simulink model "full_system"  (R2022b)
settings: Solver=VariableStepAuto  StartTime=0.0  StopTime=60  RelTol=1e-3
model workspace (MAT data in the model file):
  J_left = Simulink.Parameter
  J_left.Value = 0.0896732223267
  J_left.Description = 'left wheel inertia'
  J_left.DataType = 'auto'
  J_left.Complexity = 'real'
  J_left.Dimensions = [1 1]
  J_right = Simulink.Parameter
  J_right.Value = 0.0740595319322
  J_right.Description = 'right wheel inertia'
  J_right.DataType = 'auto'
  J_right.Complexity = 'real'
  J_right.Dimensions = [1 1]
  K_L = Simulink.Parameter
  K_L.Value = Simulink.data.Expression
  K_L.Value.ExpressionString = "1.2108*K_R"
  K_L.DataType = 'auto'
  K_L.Complexity = 'real'
  K_L.Dimensions = -1
  K_R = Simulink.Parameter
  K_R.Value = 2.0947
  K_R.DataType = 'auto'
  K_R.Complexity = 'real'
  K_R.Dimensions = [1 1]
  K_w = Simulink.Parameter
  K_w.Value = 4
  K_w.Description = 'heading controller gain'
  K_w.DataType = 'auto'
  K_w.Complexity = 'real'
  K_w.Dimensions = [1 1]
  T_max = Simulink.Parameter
  T_max.Value = 10
  T_max.Description = 'maximum allowable torque command'
  T_max.DataType = 'auto'
  T_max.DocUnits = 'N*m'
  T_max.Complexity = 'real'
  T_max.Dimensions = [1 1]
  bw = Simulink.Parameter
  bw.Value = 0.24
  bw.Description = 'Distance between the two drive wheels'
  bw.DataType = 'auto'
  bw.DocUnits = 'm'
  bw.Complexity = 'real'
  bw.Dimensions = [1 1]
  r_turn = Simulink.Parameter
  r_turn.Value = 0.2
  r_turn.Description = 'Minimum turn radius of the car'
  r_turn.DataType = 'auto'
  r_turn.Min = 0
  r_turn.DocUnits = 'm'
  r_turn.Complexity = 'real'
  r_turn.Dimensions = [1 1]
  r_wheel = Simulink.Parameter
  r_wheel.Value = 0.11
  r_wheel.Description = 'Wheel radius'
  r_wheel.DataType = 'auto'
  r_wheel.DocUnits = 'm'
  r_wheel.Complexity = 'real'
  r_wheel.Dimensions = [1 1]
  v_base = Simulink.Parameter
  v_base.Value = 0.8
  v_base.Description = 'base wheel speed (m/s) used for turns
    | v_base = w_turn_max * bw/2'
  v_base.DataType = 'auto'
  v_base.DocUnits = 'm/s'
  v_base.Complexity = 'real'
  v_base.Dimensions = [1 1]
  v_max = Simulink.Parameter
  v_max.Value = 1
  v_max.Description = 'max car speed in m/s'
  v_max.DataType = 'auto'
  v_max.DocUnits = 'm/s'
  v_max.Complexity = 'real'
  v_max.Dimensions = [1 1]
  w_max = Simulink.Parameter
  w_max.Value = Simulink.data.Expression
  w_max.Value.ExpressionString = "9.0909*v_max"
  w_max.Description = 'max wheel speed in rad/s
    | w_max = v_max/r_wheel'
  w_max.DataType = 'auto'
  w_max.DocUnits = 'rad/s'
  w_max.Complexity = 'real'
  w_max.Dimensions = -1
  w_turn_max = Simulink.Parameter
  w_turn_max.Value = 4
  w_turn_max.Description = 'max turning speed of car in rad/s
    | w_turn_max = w_max * r_wheel/bw'
  w_turn_max.DataType = 'auto'
  w_turn_max.DocUnits = 'rad/s'
  w_turn_max.Complexity = 'real'
  w_turn_max.Dimensions = [1 1]
values from neighbouring files (symbols this model uses):
  J_left = 0.089673222326686    (= 0.0896732223267)    [calc_torque_gains.m]
  J_right = 0.074059531932167    (= 0.0740595319322)    [calc_torque_gains.m]
undefined symbols (not defined in the file or in its folder): duration, effort, index, joint_name, K_l, K_r, left_wheel_hinge, model_name, pioneer2dx, right_wheel_hinge
libraries: robotgazebolib x46, simulink x4, robotcorelib x2, SignalEditorBlockLib x1
settings Model: Creator=22546723@sun.ac.za  LastModifiedBy=22546723@sun.ac.za

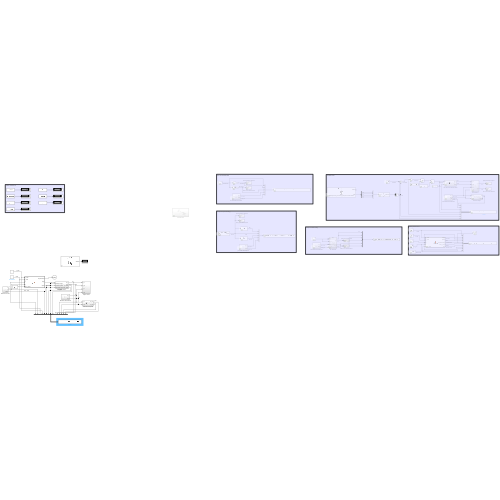
[thumbnail: Simulink's stored preview of the top-level diagram]
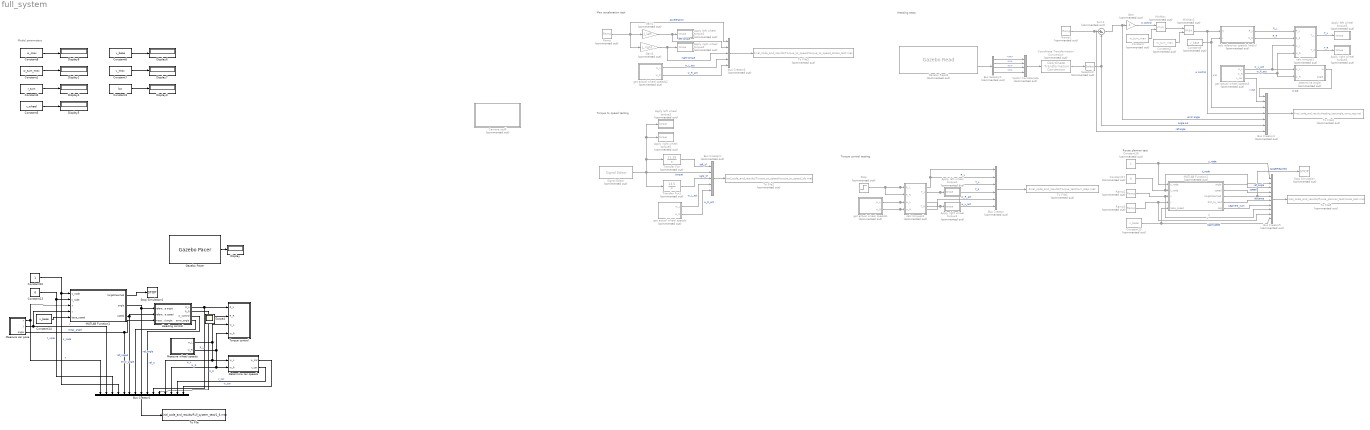
== system full_system ==
  note: Route planner test
  note: Heading tests
  note: Torque control testing
  note: Max acceleration test
  note: Torque to speed testing
  note: Model parameters
  Apply left wheel torque1 : Subsystem  Commented=on
  Apply left wheel torque2 : Subsystem  Commented=on
  Apply left wheel torque3 : Subsystem  Commented=on
  Apply left wheel torque5 : Subsystem  Commented=on
  Apply right wheel torque1 : Subsystem  Commented=on
  Apply right wheel torque2 : Subsystem  Commented=on
  Apply right wheel torque3 : Subsystem  Commented=on
  Apply right wheel torque5 : Subsystem  Commented=on
  Bus Creator : BusCreator  Commented=on  Inputs=6
  Bus Creator1 : BusCreator  Inputs=15
  Bus Creator2 : BusCreator  Commented=on  Inputs=5
  Bus Creator3 : BusCreator  Commented=on  Inputs=5
  Bus Creator4 : BusCreator  Commented=on  Inputs=7
  Bus Creator5 : BusCreator  Commented=on  Inputs=10
  Bus Selector1 : BusSelector  Commented=on  OutputSignals=orientation.w,orientation.x,orientation.y,orientation.z
  Camera stuff : Subsystem  Commented=on
  Constant : Constant  Commented=on  Value=w_turn_max
  Constant1 : Constant  Value=w_turn_max
  Constant10 : Constant
  Constant13 : Constant  Value=6
  Constant14 : Constant  Value=v_base
  Constant15 : Constant  Commented=on  Value=v_base
  Constant16 : Constant  Commented=on
  Constant17 : Constant  Commented=on  Value=8
  Constant2 : Constant  Commented=on  Value=-w_turn_max
  Constant3 : Constant  Value=bw
  Constant4 : Constant  Value=r_turn
  Constant5 : Constant  Value=r_wheel
  Constant6 : Constant  Value=v_base
  Constant7 : Constant  Value=v_max
  Constant8 : Constant  Value=w_max
  Constant9 : Constant  Commented=on  Value=v_base
  Coordinate Transformation Conversion : robotcorelib/Coordinate Transformation Conversion  Commented=on  InputRepresentation=Quaternion  InputEulerSequence=ZYX  ShowTrVecInputPort=on  OutputRepresentation=Euler Angles  OutputEulerSequence=ZYX  ShowTrVecOutputPort=on  SimulateUsing=Interpreted execution
  Determine car speeds : Subsystem
  Display{,2..8} (8 alike) : Display
  Gain : Gain  Commented=on  Gain=4
  Gain2 : Gain  Commented=on  Gain=J_left
  Gain3 : Gain  Commented=on  Gain=J_right
  Gazebo Pacer : robotgazebolib/Gazebo Pacer  ResetBehavior=Reset Gazebo simulation time  SampleTime=0.001
  Gazebo Read4 : robotgazebolib/Gazebo Read  Commented=on  topicSource=From Gazebo  topic=/gazebo/ground_truth/world_pose/pioneer2dx/chassis  messageType=gazebo_msgs/Pose  sampleTime=0.001  fixedAxisBusStatus=off  jointAxisCount=2
  Heading control : Subsystem
  MATLAB Function1 : MATLAB Function  TreatAsAtomicUnit=on
  MATLAB Function2 : MATLAB Function  Commented=on  TreatAsAtomicUnit=on
  Measure car pose : Subsystem
  Measure wheel speeds : Subsystem
  MinMax : MinMax  Commented=on  Inputs=2
  MinMax1 : MinMax  Commented=on  Function=max  Inputs=2
  Ramp : simulink/Sources/Ramp  Commented=on  slope=1  start=0  InitialOutput=0
  Ramp1 : simulink/Sources/Ramp  Commented=on  slope=-1  start=0  InitialOutput=0
  Ramp2 : simulink/Sources/Ramp  Commented=on  slope=8/16.7  start=0  InitialOutput=0
  Ramp3 : simulink/Sources/Ramp  Commented=on  slope=1/16.7  start=0  InitialOutput=0
  Selector2 : Selector  Commented=on  InputPortWidth=3  IndexOptions=Index vector (dialog)  Indices=1  OutputSizes=1
  Signal Editor : SignalEditorBlockLib/Signal Editor  Commented=on  FileName=test_signals.mat  ActiveScenario=torque_to_speed  ActiveSignal=torque  IsBus=off  OutputBusObjectStr=Bus: BusObject  SampleTime=0  Interpolate=off  ZeroCross=off  OutputAfterFinalValue=Setting to zero  Unit=inherit  PreserveSignalName=on
  Step : Step  Commented=on  Time=0  After=4  SampleTime=0
  Stop Simulation : Stop  Commented=on
  Stop Simulation1 : Stop
  Sum1 : Sum  Commented=on  Inputs=|+-
  To File : ToFile  Filename=Final_code_and_results/Full_system_test/1_6.mat  MatrixName=data  SaveFormat=Timeseries
  To File1 : ToFile  Commented=on  Filename=Final_code_and_results/Torque_test/turn_step.mat  MatrixName=data  SaveFormat=Timeseries
  To File2 : ToFile  Commented=on  Filename=Final_code_and_results/Torque_to_speed/torque_to_speed_tfs.mat  MatrixName=data  SaveFormat=Timeseries
  To File3 : ToFile  Commented=on  Filename=Final_code_and_results/Torque_to_speed/torque_to_speed_stress_test.mat  MatrixName=data  SaveFormat=Timeseries
  To File4 : ToFile  Commented=on  Filename=Final_code_and_results/Heading_test/angle_ramp_neg.mat  MatrixName=data  SaveFormat=Timeseries
  To File5 : ToFile  Commented=on  Filename=Final_code_and_results/Route_planner_test/route_test.mat  MatrixName=data  SaveFormat=Timeseries
  Torque control : Subsystem
  Transfer Fcn : TransferFcn  Commented=on  Numerator=11.15  Denominator=[1 0]
  Transfer Fcn1 : TransferFcn  Commented=on  Numerator=13.5  Denominator=[1 0]
  Vector Concatenate : Concatenate  Commented=on  NumInputs=4
  calc reference speeds (rad/s) : Subsystem  Commented=on
  calc torques1 : Subsystem  Commented=on
  calc torques3 : Subsystem  Commented=on
  determine angle : Subsystem  Commented=on
  get actual wheel speeds : Subsystem  Commented=on
  get actual wheel speeds1 : Subsystem  Commented=on
  get actual wheel speeds2 : Subsystem  Commented=on
  get actual wheel speeds3 : Subsystem  Commented=on
  Scope4 : Scope
  wires:
  Gazebo Pacer/1 -> Display/1
  Constant1/1 -> Display2/1
  Constant3/1 -> Display3/1
  Constant4/1 -> Display4/1
  Constant5/1 -> Display5/1
  Constant6/1 -> Display6/1
  Constant7/1 -> Display7/1
  Constant8/1 -> Display8/1
  Constant10/1 -> MATLAB Function1/1(s_node), Bus Creator1/4  "s_node"
  Constant13/1 -> MATLAB Function1/2(t_node), Bus Creator1/3  "t_node"
  Constant14/1 -> MATLAB Function1/5(base_speed)
  Signal Editor/1 -> Apply left wheel torque5/1(torque), Apply right wheel torque5/1(torque), Transfer Fcn/1, Bus Creator2/2, Transfer Fcn1/1  "torque"
  Bus Creator2/1 -> To File2/1
  Transfer Fcn/1 -> Bus Creator2/1  "left_tf"
  Transfer Fcn1/1 -> Bus Creator2/3  "right_tf"
  get actual wheel speeds/1(w_L) -> Bus Creator2/4  "w_L_act"
  get actual wheel speeds/2(w_R) -> Bus Creator2/5  "w_R_act"
  get actual wheel speeds1/1(w_L) -> Bus Creator/6, calc torques3/3(w_L)  "w_L_act"
  get actual wheel speeds1/2(w_R) -> Bus Creator/5, calc torques3/4(w_R)  "w_R_act"
  calc torques3/2(T_R) -> Bus Creator/4, Apply right wheel torque1/1(torque)  "T_R"
  calc torques3/1(T_L) -> Bus Creator/3, Apply left wheel torque1/1(torque)  "T_L"
  Step/1 -> Bus Creator/1, Bus Creator/2, calc torques3/1(R_L), calc torques3/2(R_R)  "R_L"
  Bus Creator/1 -> To File1/1
  Gain3/1 -> Apply right wheel torque2/1(torque), Bus Creator3/3  "right torque"
  Gain2/1 -> Apply left wheel torque2/1(torque), Bus Creator3/2  "left torque"
  Ramp/1 -> Gain3/1, Gain2/1, Bus Creator3/1  "acceleration"
  get actual wheel speeds2/2(w_R) -> Bus Creator3/5  "w_R_act"
  get actual wheel speeds2/1(w_L) -> Bus Creator3/4  "w_L_act"
  Bus Creator3/1 -> To File3/1
  Gain/1 -> MinMax/1  "w control"
  Constant2/1 -> MinMax1/2
  MinMax/1 -> MinMax1/1
  Constant/1 -> MinMax/2
  Sum1/1 -> Bus Creator4/5, Gain/1  "error angle"
  Selector2/1 -> Bus Creator4/6, Sum1/2  "angle out"
  Gazebo Read4/2 -> Bus Selector1/1
  Coordinate Transformation Conversion/1 -> Selector2/1
  Bus Selector1/4 -> Vector Concatenate/4  "<z>"
  Bus Selector1/3 -> Vector Concatenate/3  "<y>"
  Bus Selector1/1 -> Vector Concatenate/1  "<w>"
  Bus Selector1/2 -> Vector Concatenate/2  "<x>"
  Vector Concatenate/1 -> Coordinate Transformation Conversion/1
  get actual wheel speeds3/1(w_L) -> determine angle/1(w_L), calc torques1/3(w_L)  "w_L_act"
  calc reference speeds (rad/s)/1(R_L) -> calc torques1/1(R_L)  "R_L"
  calc reference speeds (rad/s)/2(R_R) -> calc torques1/2(R_R)  "R_R"
  Ramp1/1 -> Bus Creator4/7, Sum1/1  "ref angle"
  calc torques1/2(T_R) -> Apply right wheel torque3/1(torque)  "T_R"
  MinMax1/1 -> calc reference speeds (rad/s)/1(w), Bus Creator4/4  "w control"
  get actual wheel speeds3/2(w_R) -> determine angle/2(w_R), calc torques1/4(w_R)  "w_R_act"
  calc torques1/1(T_L) -> Apply left wheel torque3/1(torque)  "T_L"
  Constant9/1 -> Bus Creator4/3, calc reference speeds (rad/s)/2(v)  "v in"
  Bus Creator4/1 -> To File4/1
  determine angle/1(w) -> Bus Creator4/1  "w out"
  get actual wheel speeds3/3(v_car) -> Bus Creator4/2  "v out"
  Constant15/1 -> MATLAB Function2/5(base_speed), Bus Creator5/10  "base speed"
  Ramp3/1 -> MATLAB Function2/4(y), Bus Creator5/9  "y"
  Ramp2/1 -> Bus Creator5/8, MATLAB Function2/3(x)  "x"
  Constant17/1 -> Bus Creator5/2, MATLAB Function2/2(t_node)  "t_node"
  Constant16/1 -> MATLAB Function2/1(s_node), Bus Creator5/1  "s_node"
  MATLAB Function2/1(angle) -> Bus Creator5/3  "ref_angle"
  MATLAB Function2/2(speed) -> Bus Creator5/4  "speed"
  MATLAB Function2/3(targetReached) -> Bus Creator5/5, Stop Simulation/1  "targetReached"
  MATLAB Function2/4(dist_to_next) -> Bus Creator5/6  "distance"
  MATLAB Function2/5(seg) -> Bus Creator5/7  "segment_num"
  Bus Creator5/1 -> To File5/1
  MATLAB Function1/1(targetReached) -> Stop Simulation1/1
  Measure wheel speeds/1(w_L) -> Bus Creator1/12, Determine car speeds/1(w_L), Torque control/3(w_L)  "w_L"
  Measure wheel speeds/2(w_R) -> Bus Creator1/13, Determine car speeds/2(w_R), Torque control/4(w_R)  "w_R"
  MATLAB Function1/2(angle) -> Heading control/1(reference angle), Bus Creator1/8  "ref_angle"
  MATLAB Function1/3(speed) -> Heading control/2(reference speed), Bus Creator1/6  "ref_speed"
  Heading control/1(R_L) -> Bus Creator1/10, Torque control/1(R_L)  "R_L"
  Heading control/2(R_R) -> Bus Creator1/11, Torque control/2(R_R)  "R_R"
  Measure car pose/3(angle) -> Heading control/3(measured angle), Bus Creator1/5  "meas_angle"
  Measure car pose/1(x) -> MATLAB Function1/3(x), Bus Creator1/1  "x"
  Measure car pose/2(y) -> MATLAB Function1/4(y), Bus Creator1/2  "y"
  Determine car speeds/1(w_car) -> Bus Creator1/15  "w_car"
  Determine car speeds/2(v_car) -> Bus Creator1/14  "v_car"
  Bus Creator1/1 -> To File/1
  Heading control/3(w_control) -> Bus Creator1/9  "ref_w"
  Heading control/4(error_angle) -> Bus Creator1/7  "error_angle"

== system full_system/Apply left wheel torque1 ==
  torque : Inport  SampleTime=0.001
  Bus Assignment : BusAssignment  AssignedSignals=model_name,joint_name,index,effort,duration.nano_seconds
  Constant : Constant  Value=0  OutDataTypeStr=uint32  SampleTime=0.001
  Constant1 : Constant  Value=1e7  SampleTime=0.001
  Gazebo Apply Command : robotgazebolib/Gazebo Apply Command  cmdType=ApplyJointTorque  sampleTime=0.001
  Gazebo Blank Message : robotgazebolib/Gazebo Blank Message  msgType=ApplyJointTorque  sampleTime=0.001  busName='Gazebo_SL_Bus_gazebo_msgs_ApplyJointTorque'
  Gazebo Select Entity : robotgazebolib/Gazebo Select Entity  modelElemName=pioneer2dx/left_wheel_hinge  outputArraySize=128  OutputLabel=Joint  SelectType=Joint
  wires:
  Gazebo Select Entity/1 -> Bus Assignment/2
  Bus Assignment/1 -> Gazebo Apply Command/1
  Gazebo Blank Message/1 -> Bus Assignment/1
  Constant/1 -> Bus Assignment/4
  Gazebo Select Entity/2 -> Bus Assignment/3
  Constant1/1 -> Bus Assignment/6
  torque/1 -> Bus Assignment/5

== system full_system/Apply left wheel torque2 ==
  torque : Inport  SampleTime=0.001
  Bus Assignment : BusAssignment  AssignedSignals=model_name,joint_name,index,effort,duration.nano_seconds
  Constant : Constant  Value=0  OutDataTypeStr=uint32  SampleTime=0.001
  Constant1 : Constant  Value=1e7  SampleTime=0.001
  Gazebo Apply Command : robotgazebolib/Gazebo Apply Command  cmdType=ApplyJointTorque  sampleTime=0.001
  Gazebo Blank Message : robotgazebolib/Gazebo Blank Message  msgType=ApplyJointTorque  sampleTime=0.001  busName='Gazebo_SL_Bus_gazebo_msgs_ApplyJointTorque'
  Gazebo Select Entity : robotgazebolib/Gazebo Select Entity  modelElemName=pioneer2dx/left_wheel_hinge  outputArraySize=128  OutputLabel=Joint  SelectType=Joint
  wires:
  Gazebo Select Entity/1 -> Bus Assignment/2
  Bus Assignment/1 -> Gazebo Apply Command/1
  Gazebo Blank Message/1 -> Bus Assignment/1
  Constant/1 -> Bus Assignment/4
  Gazebo Select Entity/2 -> Bus Assignment/3
  Constant1/1 -> Bus Assignment/6
  torque/1 -> Bus Assignment/5

== system full_system/Apply left wheel torque3 ==
  torque : Inport  SampleTime=0.001
  Bus Assignment : BusAssignment  AssignedSignals=model_name,joint_name,index,effort,duration.nano_seconds
  Constant : Constant  Value=0  OutDataTypeStr=uint32  SampleTime=0.001
  Constant1 : Constant  Value=1e7  SampleTime=0.001
  Gazebo Apply Command : robotgazebolib/Gazebo Apply Command  cmdType=ApplyJointTorque  sampleTime=0.001
  Gazebo Blank Message : robotgazebolib/Gazebo Blank Message  msgType=ApplyJointTorque  sampleTime=0.001  busName='Gazebo_SL_Bus_gazebo_msgs_ApplyJointTorque'
  Gazebo Select Entity : robotgazebolib/Gazebo Select Entity  modelElemName=pioneer2dx/left_wheel_hinge  outputArraySize=128  OutputLabel=Joint  SelectType=Joint
  wires:
  Gazebo Select Entity/1 -> Bus Assignment/2
  Bus Assignment/1 -> Gazebo Apply Command/1
  Gazebo Blank Message/1 -> Bus Assignment/1
  Constant/1 -> Bus Assignment/4
  Gazebo Select Entity/2 -> Bus Assignment/3
  Constant1/1 -> Bus Assignment/6
  torque/1 -> Bus Assignment/5

== system full_system/Apply left wheel torque5 ==
  torque : Inport  SampleTime=0.001
  Bus Assignment : BusAssignment  AssignedSignals=model_name,joint_name,index,effort,duration.nano_seconds
  Constant : Constant  Value=0  OutDataTypeStr=uint32  SampleTime=0.001
  Constant1 : Constant  Value=1e7  SampleTime=0.001
  Gazebo Apply Command : robotgazebolib/Gazebo Apply Command  cmdType=ApplyJointTorque  sampleTime=0.001
  Gazebo Blank Message : robotgazebolib/Gazebo Blank Message  msgType=ApplyJointTorque  sampleTime=0.001  busName='Gazebo_SL_Bus_gazebo_msgs_ApplyJointTorque'
  Gazebo Select Entity : robotgazebolib/Gazebo Select Entity  modelElemName=pioneer2dx/left_wheel_hinge  outputArraySize=128  OutputLabel=Joint  SelectType=Joint
  wires:
  Gazebo Select Entity/1 -> Bus Assignment/2
  Bus Assignment/1 -> Gazebo Apply Command/1
  Gazebo Blank Message/1 -> Bus Assignment/1
  Constant/1 -> Bus Assignment/4
  Gazebo Select Entity/2 -> Bus Assignment/3
  Constant1/1 -> Bus Assignment/6
  torque/1 -> Bus Assignment/5

== system full_system/Apply right wheel torque1 ==
  torque : Inport  SampleTime=0.001
  Bus Assignment : BusAssignment  AssignedSignals=model_name,joint_name,index,effort,duration.nano_seconds
  Constant : Constant  Value=0  OutDataTypeStr=uint32  SampleTime=0.001
  Constant1 : Constant  Value=1e7  SampleTime=0.001
  Gazebo Apply Command : robotgazebolib/Gazebo Apply Command  cmdType=ApplyJointTorque  sampleTime=0.001
  Gazebo Blank Message : robotgazebolib/Gazebo Blank Message  msgType=ApplyJointTorque  sampleTime=0.001  busName='Gazebo_SL_Bus_gazebo_msgs_ApplyJointTorque'
  Gazebo Select Entity : robotgazebolib/Gazebo Select Entity  modelElemName=pioneer2dx/right_wheel_hinge  outputArraySize=128  OutputLabel=Joint  SelectType=Joint
  wires:
  Gazebo Select Entity/1 -> Bus Assignment/2
  Bus Assignment/1 -> Gazebo Apply Command/1
  Gazebo Blank Message/1 -> Bus Assignment/1
  Constant/1 -> Bus Assignment/4
  Gazebo Select Entity/2 -> Bus Assignment/3
  Constant1/1 -> Bus Assignment/6
  torque/1 -> Bus Assignment/5

== system full_system/Apply right wheel torque2 ==
  torque : Inport  SampleTime=0.001
  Bus Assignment : BusAssignment  AssignedSignals=model_name,joint_name,index,effort,duration.nano_seconds
  Constant : Constant  Value=0  OutDataTypeStr=uint32  SampleTime=0.001
  Constant1 : Constant  Value=1e7  SampleTime=0.001
  Gazebo Apply Command : robotgazebolib/Gazebo Apply Command  cmdType=ApplyJointTorque  sampleTime=0.001
  Gazebo Blank Message : robotgazebolib/Gazebo Blank Message  msgType=ApplyJointTorque  sampleTime=0.001  busName='Gazebo_SL_Bus_gazebo_msgs_ApplyJointTorque'
  Gazebo Select Entity : robotgazebolib/Gazebo Select Entity  modelElemName=pioneer2dx/right_wheel_hinge  outputArraySize=128  OutputLabel=Joint  SelectType=Joint
  wires:
  Gazebo Select Entity/1 -> Bus Assignment/2
  Bus Assignment/1 -> Gazebo Apply Command/1
  Gazebo Blank Message/1 -> Bus Assignment/1
  Constant/1 -> Bus Assignment/4
  Gazebo Select Entity/2 -> Bus Assignment/3
  Constant1/1 -> Bus Assignment/6
  torque/1 -> Bus Assignment/5

== system full_system/Apply right wheel torque3 ==
  torque : Inport  SampleTime=0.001
  Bus Assignment : BusAssignment  AssignedSignals=model_name,joint_name,index,effort,duration.nano_seconds
  Constant : Constant  Value=0  OutDataTypeStr=uint32  SampleTime=0.001
  Constant1 : Constant  Value=1e7  SampleTime=0.001
  Gazebo Apply Command : robotgazebolib/Gazebo Apply Command  cmdType=ApplyJointTorque  sampleTime=0.001
  Gazebo Blank Message : robotgazebolib/Gazebo Blank Message  msgType=ApplyJointTorque  sampleTime=0.001  busName='Gazebo_SL_Bus_gazebo_msgs_ApplyJointTorque'
  Gazebo Select Entity : robotgazebolib/Gazebo Select Entity  modelElemName=pioneer2dx/right_wheel_hinge  outputArraySize=128  OutputLabel=Joint  SelectType=Joint
  wires:
  Gazebo Select Entity/1 -> Bus Assignment/2
  Bus Assignment/1 -> Gazebo Apply Command/1
  Gazebo Blank Message/1 -> Bus Assignment/1
  Constant/1 -> Bus Assignment/4
  Gazebo Select Entity/2 -> Bus Assignment/3
  Constant1/1 -> Bus Assignment/6
  torque/1 -> Bus Assignment/5

== system full_system/Apply right wheel torque5 ==
  torque : Inport  SampleTime=0.001
  Bus Assignment : BusAssignment  AssignedSignals=model_name,joint_name,index,effort,duration.nano_seconds
  Constant : Constant  Value=0  OutDataTypeStr=uint32  SampleTime=0.001
  Constant1 : Constant  Value=1e7  SampleTime=0.001
  Gazebo Apply Command : robotgazebolib/Gazebo Apply Command  cmdType=ApplyJointTorque  sampleTime=0.001
  Gazebo Blank Message : robotgazebolib/Gazebo Blank Message  msgType=ApplyJointTorque  sampleTime=0.001  busName='Gazebo_SL_Bus_gazebo_msgs_ApplyJointTorque'
  Gazebo Select Entity : robotgazebolib/Gazebo Select Entity  modelElemName=pioneer2dx/right_wheel_hinge  outputArraySize=128  OutputLabel=Joint  SelectType=Joint
  wires:
  Gazebo Select Entity/1 -> Bus Assignment/2
  Bus Assignment/1 -> Gazebo Apply Command/1
  Gazebo Blank Message/1 -> Bus Assignment/1
  Constant/1 -> Bus Assignment/4
  Gazebo Select Entity/2 -> Bus Assignment/3
  Constant1/1 -> Bus Assignment/6
  torque/1 -> Bus Assignment/5

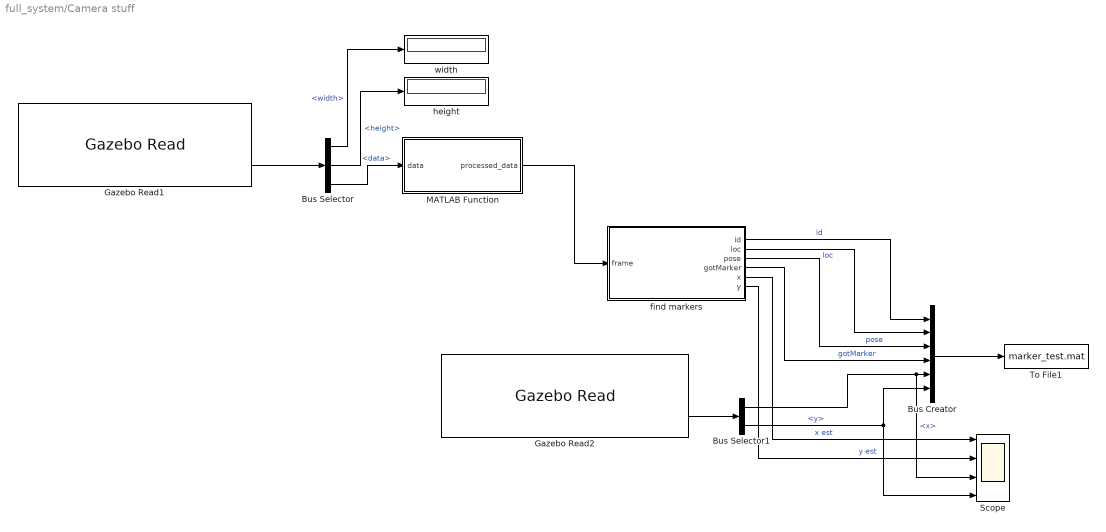
== system full_system/Camera stuff ==
  Bus Creator : BusCreator  Inputs=6
  Bus Selector : BusSelector  OutputSignals=width,height,data
  Bus Selector1 : BusSelector  OutputSignals=position.x,position.y
  Gazebo Read1 : robotgazebolib/Gazebo Read  topicSource=From Gazebo  topic=/gazebo/default/pioneer2dx/camera/camera/image  messageType=gazebo_msgs/Image  sampleTime=0.001  fixedAxisBusStatus=off  jointAxisCount=2
  Gazebo Read2 : robotgazebolib/Gazebo Read  topicSource=From Gazebo  topic=/gazebo/ground_truth/world_pose/pioneer2dx/camera  messageType=gazebo_msgs/Pose  sampleTime=0.001  fixedAxisBusStatus=off  jointAxisCount=2
  MATLAB Function : MATLAB Function  TreatAsAtomicUnit=on
  Scope : Scope  NumInputPorts=4
  To File1 : ToFile  Filename=marker_test.mat  MatrixName=data  SaveFormat=Timeseries
  find markers : MATLAB Function  TreatAsAtomicUnit=on
  height : Display
  width : Display
  wires:
  Bus Creator/1 -> To File1/1
  find markers/3(pose) -> Bus Creator/3  "pose"
  find markers/1(id) -> Bus Creator/1  "id"
  Gazebo Read2/2 -> Bus Selector1/1
  Bus Selector/1 -> width/1  "<width>"
  find markers/6(y) -> Scope/2  "y est"
  find markers/5(x) -> Scope/1  "x est"
  Bus Selector/3 -> MATLAB Function/1(data)  "<data>"
  Bus Selector1/2 -> Scope/4, Bus Creator/6  "<y>"
  find markers/2(loc) -> Bus Creator/2  "loc"
  find markers/4(gotMarker) -> Bus Creator/4  "gotMarker"
  Gazebo Read1/2 -> Bus Selector/1
  Bus Selector/2 -> height/1  "<height>"
  Bus Selector1/1 -> Scope/3, Bus Creator/5  "<x>"
  MATLAB Function/1(processed_data) -> find markers/1(frame)

== system full_system/Determine car speeds ==
  w_L : Inport
  w_R : Inport  Port=2
  Gain2 : Gain  Gain=0.5*r_wheel
  Gain3 : Gain  Gain=r_wheel/bw
  Sum : Sum  Inputs=++|
  Sum4 : Sum  Inputs=|-+
  w_car : Outport
  v_car : Outport  Port=2
  wires:
  Gain3/1 -> w_car/1  "w_turn"
  Sum4/1 -> Gain3/1
  w_R/1 -> Sum4/2, Sum/1
  w_L/1 -> Sum4/1, Sum/2
  Gain2/1 -> v_car/1
  Sum/1 -> Gain2/1

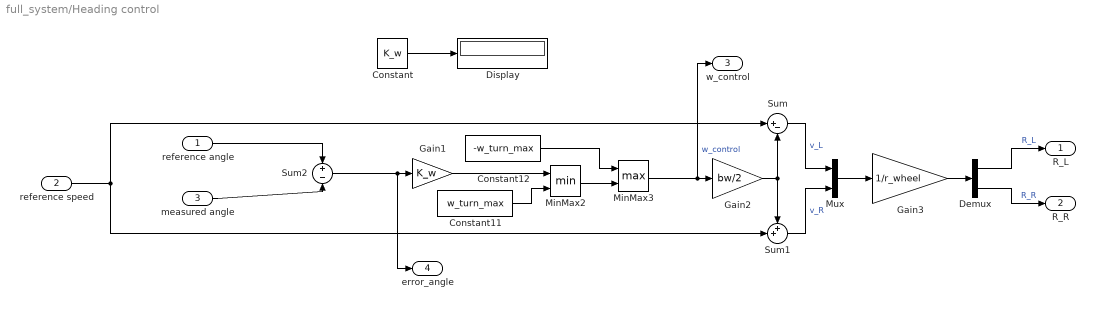
== system full_system/Heading control ==
  reference angle : Inport
  reference speed : Inport  Port=2
  measured angle : Inport  Port=3
  Constant : Constant  Value=K_w
  Constant11 : Constant  Value=w_turn_max
  Constant12 : Constant  Value=-w_turn_max
  Demux : Demux  Outputs=2
  Display : Display
  Gain1 : Gain  Gain=K_w
  Gain2 : Gain  Gain=bw/2
  Gain3 : Gain  Gain=1/r_wheel
  MinMax2 : MinMax  Inputs=2
  MinMax3 : MinMax  Function=max  Inputs=2
  Mux : Mux  Inputs=2
  Sum : Sum  Inputs=|+-
  Sum1 : Sum  Inputs=++|
  Sum2 : Sum  Inputs=+|-
  R_L : Outport
  R_R : Outport  Port=2
  w_control : Outport  Port=3
  error_angle : Outport  Port=4
  wires:
  Constant11/1 -> MinMax2/2
  Demux/2 -> R_R/1  "R_R"
  Constant12/1 -> MinMax3/1
  Gain1/1 -> MinMax2/1
  Demux/1 -> R_L/1  "R_L"
  MinMax2/1 -> MinMax3/2
  MinMax3/1 -> w_control/1, Gain2/1  "w_control"
  Mux/1 -> Gain3/1
  Gain3/1 -> Demux/1
  Sum1/1 -> Mux/2  "v_R"
  Gain2/1 -> Sum1/1, Sum/2
  Sum/1 -> Mux/1  "v_L"
  reference speed/1 -> Sum/1, Sum1/2
  Constant/1 -> Display/1
  Sum2/1 -> error_angle/1, Gain1/1
  reference angle/1 -> Sum2/1
  measured angle/1 -> Sum2/2

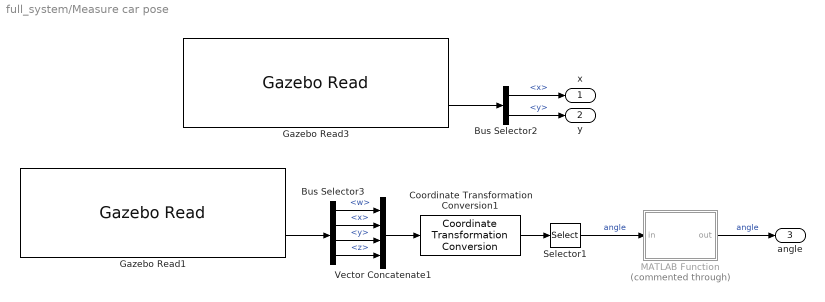
== system full_system/Measure car pose ==
  Bus Selector2 : BusSelector  OutputSignals=position.x,position.y
  Bus Selector3 : BusSelector  OutputSignals=orientation.w,orientation.x,orientation.y,orientation.z
  Coordinate Transformation Conversion1 : robotcorelib/Coordinate Transformation Conversion  InputRepresentation=Quaternion  InputEulerSequence=ZYX  ShowTrVecInputPort=on  OutputRepresentation=Euler Angles  OutputEulerSequence=ZYX  ShowTrVecOutputPort=on  SimulateUsing=Interpreted execution
  Gazebo Read1 : robotgazebolib/Gazebo Read  topicSource=From Gazebo  topic=/gazebo/ground_truth/world_pose/pioneer2dx/chassis  messageType=gazebo_msgs/Pose  sampleTime=0.001  fixedAxisBusStatus=off  jointAxisCount=2
  Gazebo Read3 : robotgazebolib/Gazebo Read  topicSource=From Gazebo  topic=/gazebo/ground_truth/world_pose/pioneer2dx/chassis  messageType=gazebo_msgs/Pose  sampleTime=0.001  fixedAxisBusStatus=off  jointAxisCount=2
  MATLAB Function : MATLAB Function  Commented=through  TreatAsAtomicUnit=on
  Selector1 : Selector  InputPortWidth=3  IndexOptions=Index vector (dialog)  Indices=1  OutputSizes=1
  Vector Concatenate1 : Concatenate  NumInputs=4
  x : Outport
  y : Outport  Port=2
  angle : Outport  Port=3
  wires:
  Coordinate Transformation Conversion1/1 -> Selector1/1
  Vector Concatenate1/1 -> Coordinate Transformation Conversion1/1
  MATLAB Function/1(out) -> angle/1  "angle"
  Bus Selector3/2 -> Vector Concatenate1/2  "<x>"
  Bus Selector2/2 -> y/1  "<y>"
  Bus Selector3/4 -> Vector Concatenate1/4  "<z>"
  Gazebo Read1/2 -> Bus Selector3/1
  Bus Selector3/1 -> Vector Concatenate1/1  "<w>"
  Gazebo Read3/2 -> Bus Selector2/1
  Bus Selector3/3 -> Vector Concatenate1/3  "<y>"
  Bus Selector2/1 -> x/1  "<x>"
  Selector1/1 -> MATLAB Function/1(in)  "angle"

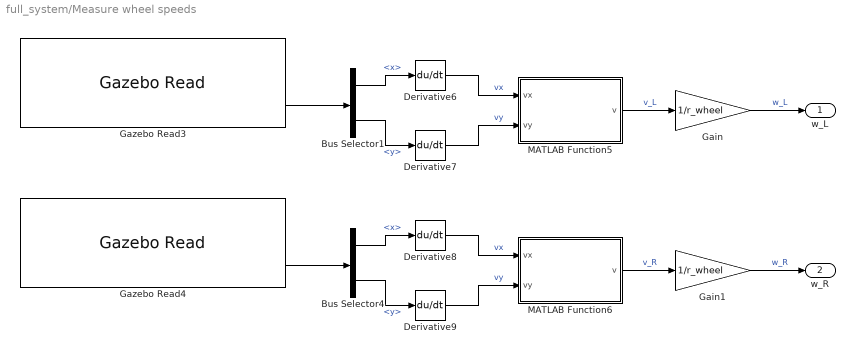
== system full_system/Measure wheel speeds ==
  Bus Selector1 : BusSelector  OutputSignals=position.x,position.y
  Bus Selector4 : BusSelector  OutputSignals=position.x,position.y
  Derivative{6..9} (4 alike) : Derivative
  Gain : Gain  Gain=1/r_wheel
  Gain1 : Gain  Gain=1/r_wheel
  Gazebo Read3 : robotgazebolib/Gazebo Read  topicSource=From Gazebo  topic=/gazebo/ground_truth/world_pose/pioneer2dx/left_wheel  messageType=gazebo_msgs/Pose  sampleTime=0.001  fixedAxisBusStatus=off  jointAxisCount=2
  Gazebo Read4 : robotgazebolib/Gazebo Read  topicSource=From Gazebo  topic=/gazebo/ground_truth/world_pose/pioneer2dx/right_wheel  messageType=gazebo_msgs/Pose  sampleTime=0.001  fixedAxisBusStatus=off  jointAxisCount=2
  MATLAB Function5 : MATLAB Function  TreatAsAtomicUnit=on
  MATLAB Function6 : MATLAB Function  TreatAsAtomicUnit=on
  w_L : Outport
  w_R : Outport  Port=2
  wires:
  Bus Selector4/1 -> Derivative8/1  "<x>"
  Bus Selector4/2 -> Derivative9/1  "<y>"
  Derivative8/1 -> MATLAB Function6/1(vx)  "vx"
  Derivative9/1 -> MATLAB Function6/2(vy)  "vy"
  Derivative6/1 -> MATLAB Function5/1(vx)  "vx"
  Gazebo Read3/2 -> Bus Selector1/1
  Bus Selector1/1 -> Derivative6/1  "<x>"
  Bus Selector1/2 -> Derivative7/1  "<y>"
  Gazebo Read4/2 -> Bus Selector4/1
  Derivative7/1 -> MATLAB Function5/2(vy)  "vy"
  MATLAB Function5/1(v) -> Gain/1  "v_L"
  Gain/1 -> w_L/1  "w_L"
  MATLAB Function6/1(v) -> Gain1/1  "v_R"
  Gain1/1 -> w_R/1  "w_R"

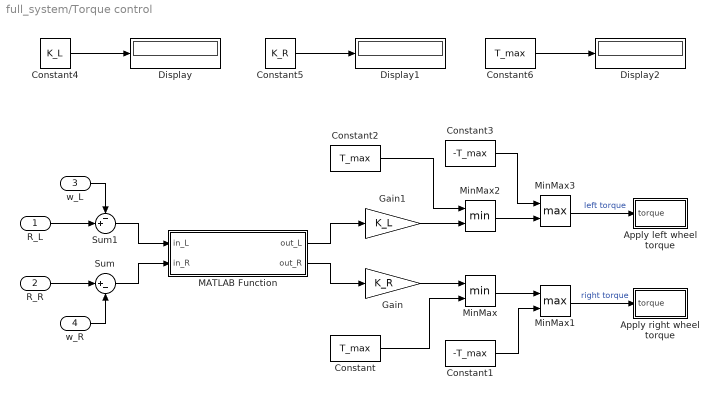
== system full_system/Torque control ==
  R_L : Inport
  R_R : Inport  Port=2
  w_L : Inport  Port=3
  w_R : Inport  Port=4
  Apply left wheel torque : Subsystem
  Apply right wheel torque : Subsystem
  Constant : Constant  Value=T_max
  Constant1 : Constant  Value=-T_max
  Constant2 : Constant  Value=T_max
  Constant3 : Constant  Value=-T_max
  Constant4 : Constant  Value=K_L
  Constant5 : Constant  Value=K_R
  Constant6 : Constant  Value=T_max
  Display : Display
  Display1 : Display
  Display2 : Display
  Gain : Gain  Gain=K_R
  Gain1 : Gain  Gain=K_L
  MATLAB Function : MATLAB Function  TreatAsAtomicUnit=on
  MinMax : MinMax  Inputs=2
  MinMax1 : MinMax  Function=max  Inputs=2
  MinMax2 : MinMax  Inputs=2
  MinMax3 : MinMax  Function=max  Inputs=2
  Sum : Sum  Inputs=|+-
  Sum1 : Sum  Inputs=-+|
  wires:
  Gain/1 -> MinMax/1
  Constant3/1 -> MinMax3/1
  Constant2/1 -> MinMax2/1
  Gain1/1 -> MinMax2/2
  R_R/1 -> Sum/1
  Constant/1 -> MinMax/2
  w_R/1 -> Sum/2
  MinMax/1 -> MinMax1/1
  MinMax1/1 -> Apply right wheel torque/1(torque)  "right torque"
  Constant1/1 -> MinMax1/2
  w_L/1 -> Sum1/1
  R_L/1 -> Sum1/2
  MinMax2/1 -> MinMax3/2
  Sum1/1 -> MATLAB Function/1(in_L)
  Sum/1 -> MATLAB Function/2(in_R)
  MATLAB Function/2(out_R) -> Gain/1
  MATLAB Function/1(out_L) -> Gain1/1
  MinMax3/1 -> Apply left wheel torque/1(torque)  "left torque"
  Constant4/1 -> Display/1
  Constant5/1 -> Display1/1
  Constant6/1 -> Display2/1

== system full_system/calc reference speeds (rad//s) ==
  w : Inport
  v : Inport  Port=2
  Demux : Demux  Outputs=2
  Gain1 : Gain  Gain=1/r_wheel
  Gain2 : Gain  Gain=bw/2
  Mux : Mux  Inputs=2
  Sum : Sum  Inputs=|+-
  Sum1 : Sum  Inputs=++|
  R_L : Outport
  R_R : Outport  Port=2
  wires:
  v/1 -> Sum/1, Sum1/2
  Sum/1 -> Mux/1
  Demux/1 -> R_L/1
  Gain2/1 -> Sum1/1, Sum/2
  Sum1/1 -> Mux/2
  Gain1/1 -> Demux/1
  Mux/1 -> Gain1/1
  w/1 -> Gain2/1
  Demux/2 -> R_R/1

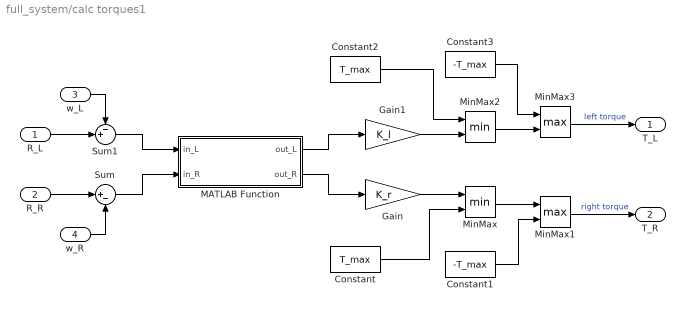
== system full_system/calc torques1 ==
  R_L : Inport
  R_R : Inport  Port=2
  w_L : Inport  Port=3
  w_R : Inport  Port=4
  Constant : Constant  Value=T_max
  Constant1 : Constant  Value=-T_max
  Constant2 : Constant  Value=T_max
  Constant3 : Constant  Value=-T_max
  Gain : Gain  Gain=K_r
  Gain1 : Gain  Gain=K_l
  MATLAB Function : MATLAB Function  TreatAsAtomicUnit=on
  MinMax : MinMax  Inputs=2
  MinMax1 : MinMax  Function=max  Inputs=2
  MinMax2 : MinMax  Inputs=2
  MinMax3 : MinMax  Function=max  Inputs=2
  Sum : Sum  Inputs=|+-
  Sum1 : Sum  Inputs=-+|
  T_L : Outport
  T_R : Outport  Port=2
  wires:
  Sum/1 -> MATLAB Function/2(in_R)
  w_R/1 -> Sum/2
  Sum1/1 -> MATLAB Function/1(in_L)
  R_R/1 -> Sum/1
  w_L/1 -> Sum1/1
  R_L/1 -> Sum1/2
  Gain/1 -> MinMax/1
  Constant/1 -> MinMax/2
  MinMax/1 -> MinMax1/1
  Constant1/1 -> MinMax1/2
  Gain1/1 -> MinMax2/2
  Constant2/1 -> MinMax2/1
  MinMax2/1 -> MinMax3/2
  Constant3/1 -> MinMax3/1
  MinMax3/1 -> T_L/1  "left torque"
  MinMax1/1 -> T_R/1  "right torque"
  MATLAB Function/1(out_L) -> Gain1/1
  MATLAB Function/2(out_R) -> Gain/1

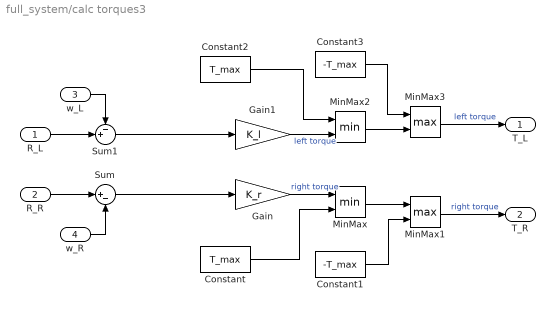
== system full_system/calc torques3 ==
  R_L : Inport
  R_R : Inport  Port=2
  w_L : Inport  Port=3
  w_R : Inport  Port=4
  Constant : Constant  Value=T_max
  Constant1 : Constant  Value=-T_max
  Constant2 : Constant  Value=T_max
  Constant3 : Constant  Value=-T_max
  Gain : Gain  Gain=K_r
  Gain1 : Gain  Gain=K_l
  MinMax : MinMax  Inputs=2
  MinMax1 : MinMax  Function=max  Inputs=2
  MinMax2 : MinMax  Inputs=2
  MinMax3 : MinMax  Function=max  Inputs=2
  Sum : Sum  Inputs=|+-
  Sum1 : Sum  Inputs=-+|
  T_L : Outport
  T_R : Outport  Port=2
  wires:
  Sum/1 -> Gain/1
  w_R/1 -> Sum/2
  Sum1/1 -> Gain1/1
  R_R/1 -> Sum/1
  w_L/1 -> Sum1/1
  R_L/1 -> Sum1/2
  Constant/1 -> MinMax/2
  MinMax/1 -> MinMax1/1
  Constant1/1 -> MinMax1/2
  Constant2/1 -> MinMax2/1
  MinMax2/1 -> MinMax3/2
  Constant3/1 -> MinMax3/1
  Gain1/1 -> MinMax2/2  "left torque"
  Gain/1 -> MinMax/1  "right torque"
  MinMax3/1 -> T_L/1  "left torque"
  MinMax1/1 -> T_R/1  "right torque"

== system full_system/determine angle ==
  w_L : Inport
  w_R : Inport  Port=2
  Gain : Gain  Gain=1/1.03
  Gain3 : Gain  Gain=r_wheel/bw
  Integrator4 : Integrator
  Sum4 : Sum  Inputs=|-+
  w : Outport
  angle : Outport  Port=2
  wires:
  Gain3/1 -> Gain/1, Integrator4/1  "w_turn"
  Sum4/1 -> Gain3/1
  w_R/1 -> Sum4/2
  Integrator4/1 -> angle/1  "angle"
  w_L/1 -> Sum4/1
  Gain/1 -> w/1

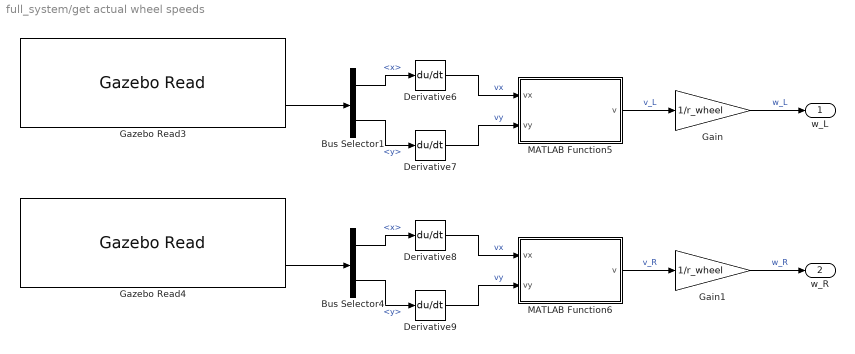
== system full_system/get actual wheel speeds ==
  Bus Selector1 : BusSelector  OutputSignals=position.x,position.y
  Bus Selector4 : BusSelector  OutputSignals=position.x,position.y
  Derivative{6..9} (4 alike) : Derivative
  Gain : Gain  Gain=1/r_wheel
  Gain1 : Gain  Gain=1/r_wheel
  Gazebo Read3 : robotgazebolib/Gazebo Read  topicSource=From Gazebo  topic=/gazebo/ground_truth/world_pose/pioneer2dx/left_wheel  messageType=gazebo_msgs/Pose  sampleTime=0.001  fixedAxisBusStatus=off  jointAxisCount=2
  Gazebo Read4 : robotgazebolib/Gazebo Read  topicSource=From Gazebo  topic=/gazebo/ground_truth/world_pose/pioneer2dx/right_wheel  messageType=gazebo_msgs/Pose  sampleTime=0.001  fixedAxisBusStatus=off  jointAxisCount=2
  MATLAB Function5 : MATLAB Function  TreatAsAtomicUnit=on
  MATLAB Function6 : MATLAB Function  TreatAsAtomicUnit=on
  w_L : Outport
  w_R : Outport  Port=2
  wires:
  Bus Selector4/1 -> Derivative8/1  "<x>"
  Bus Selector4/2 -> Derivative9/1  "<y>"
  Derivative8/1 -> MATLAB Function6/1(vx)  "vx"
  Derivative9/1 -> MATLAB Function6/2(vy)  "vy"
  Derivative6/1 -> MATLAB Function5/1(vx)  "vx"
  Gazebo Read3/2 -> Bus Selector1/1
  Bus Selector1/1 -> Derivative6/1  "<x>"
  Bus Selector1/2 -> Derivative7/1  "<y>"
  Gazebo Read4/2 -> Bus Selector4/1
  Derivative7/1 -> MATLAB Function5/2(vy)  "vy"
  MATLAB Function5/1(v) -> Gain/1  "v_L"
  Gain/1 -> w_L/1  "w_L"
  MATLAB Function6/1(v) -> Gain1/1  "v_R"
  Gain1/1 -> w_R/1  "w_R"

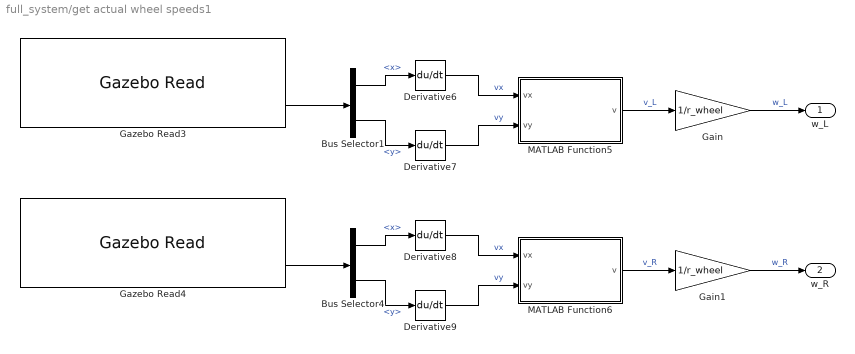
== system full_system/get actual wheel speeds1 ==
  Bus Selector1 : BusSelector  OutputSignals=position.x,position.y
  Bus Selector4 : BusSelector  OutputSignals=position.x,position.y
  Derivative{6..9} (4 alike) : Derivative
  Gain : Gain  Gain=1/r_wheel
  Gain1 : Gain  Gain=1/r_wheel
  Gazebo Read3 : robotgazebolib/Gazebo Read  topicSource=From Gazebo  topic=/gazebo/ground_truth/world_pose/pioneer2dx/left_wheel  messageType=gazebo_msgs/Pose  sampleTime=0.001  fixedAxisBusStatus=off  jointAxisCount=2
  Gazebo Read4 : robotgazebolib/Gazebo Read  topicSource=From Gazebo  topic=/gazebo/ground_truth/world_pose/pioneer2dx/right_wheel  messageType=gazebo_msgs/Pose  sampleTime=0.001  fixedAxisBusStatus=off  jointAxisCount=2
  MATLAB Function5 : MATLAB Function  TreatAsAtomicUnit=on
  MATLAB Function6 : MATLAB Function  TreatAsAtomicUnit=on
  w_L : Outport
  w_R : Outport  Port=2
  wires:
  Bus Selector4/1 -> Derivative8/1  "<x>"
  Bus Selector4/2 -> Derivative9/1  "<y>"
  Derivative8/1 -> MATLAB Function6/1(vx)  "vx"
  Derivative9/1 -> MATLAB Function6/2(vy)  "vy"
  Derivative6/1 -> MATLAB Function5/1(vx)  "vx"
  Gazebo Read3/2 -> Bus Selector1/1
  Bus Selector1/1 -> Derivative6/1  "<x>"
  Bus Selector1/2 -> Derivative7/1  "<y>"
  Gazebo Read4/2 -> Bus Selector4/1
  Derivative7/1 -> MATLAB Function5/2(vy)  "vy"
  MATLAB Function5/1(v) -> Gain/1  "v_L"
  Gain/1 -> w_L/1  "w_L"
  MATLAB Function6/1(v) -> Gain1/1  "v_R"
  Gain1/1 -> w_R/1  "w_R"

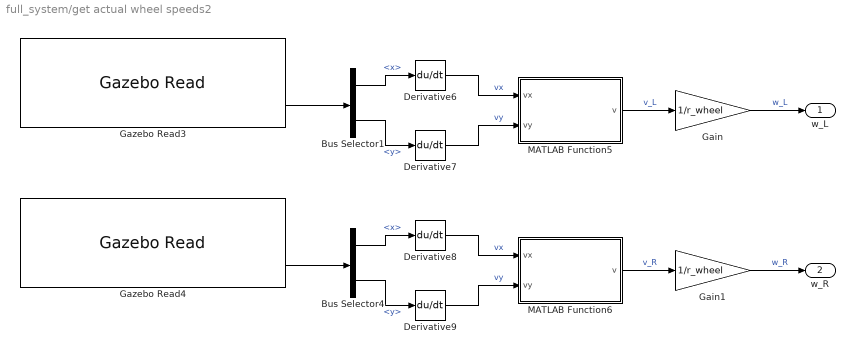
== system full_system/get actual wheel speeds2 ==
  Bus Selector1 : BusSelector  OutputSignals=position.x,position.y
  Bus Selector4 : BusSelector  OutputSignals=position.x,position.y
  Derivative{6..9} (4 alike) : Derivative
  Gain : Gain  Gain=1/r_wheel
  Gain1 : Gain  Gain=1/r_wheel
  Gazebo Read3 : robotgazebolib/Gazebo Read  topicSource=From Gazebo  topic=/gazebo/ground_truth/world_pose/pioneer2dx/left_wheel  messageType=gazebo_msgs/Pose  sampleTime=0.001  fixedAxisBusStatus=off  jointAxisCount=2
  Gazebo Read4 : robotgazebolib/Gazebo Read  topicSource=From Gazebo  topic=/gazebo/ground_truth/world_pose/pioneer2dx/right_wheel  messageType=gazebo_msgs/Pose  sampleTime=0.001  fixedAxisBusStatus=off  jointAxisCount=2
  MATLAB Function5 : MATLAB Function  TreatAsAtomicUnit=on
  MATLAB Function6 : MATLAB Function  TreatAsAtomicUnit=on
  w_L : Outport
  w_R : Outport  Port=2
  wires:
  Bus Selector4/1 -> Derivative8/1  "<x>"
  Bus Selector4/2 -> Derivative9/1  "<y>"
  Derivative8/1 -> MATLAB Function6/1(vx)  "vx"
  Derivative9/1 -> MATLAB Function6/2(vy)  "vy"
  Derivative6/1 -> MATLAB Function5/1(vx)  "vx"
  Gazebo Read3/2 -> Bus Selector1/1
  Bus Selector1/1 -> Derivative6/1  "<x>"
  Bus Selector1/2 -> Derivative7/1  "<y>"
  Gazebo Read4/2 -> Bus Selector4/1
  Derivative7/1 -> MATLAB Function5/2(vy)  "vy"
  MATLAB Function5/1(v) -> Gain/1  "v_L"
  Gain/1 -> w_L/1  "w_L"
  MATLAB Function6/1(v) -> Gain1/1  "v_R"
  Gain1/1 -> w_R/1  "w_R"

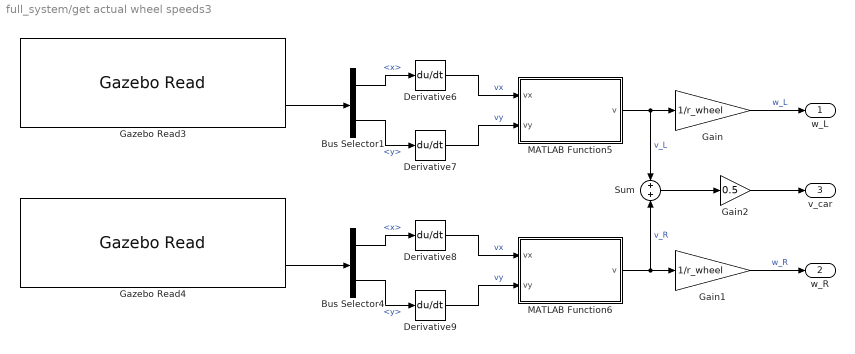
== system full_system/get actual wheel speeds3 ==
  Bus Selector1 : BusSelector  OutputSignals=position.x,position.y
  Bus Selector4 : BusSelector  OutputSignals=position.x,position.y
  Derivative{6..9} (4 alike) : Derivative
  Gain : Gain  Gain=1/r_wheel
  Gain1 : Gain  Gain=1/r_wheel
  Gain2 : Gain  Gain=0.5
  Gazebo Read3 : robotgazebolib/Gazebo Read  topicSource=From Gazebo  topic=/gazebo/ground_truth/world_pose/pioneer2dx/left_wheel  messageType=gazebo_msgs/Pose  sampleTime=0.001  fixedAxisBusStatus=off  jointAxisCount=2
  Gazebo Read4 : robotgazebolib/Gazebo Read  topicSource=From Gazebo  topic=/gazebo/ground_truth/world_pose/pioneer2dx/right_wheel  messageType=gazebo_msgs/Pose  sampleTime=0.001  fixedAxisBusStatus=off  jointAxisCount=2
  MATLAB Function5 : MATLAB Function  TreatAsAtomicUnit=on
  MATLAB Function6 : MATLAB Function  TreatAsAtomicUnit=on
  Sum : Sum  Inputs=+|+
  w_L : Outport
  w_R : Outport  Port=2
  v_car : Outport  Port=3
  wires:
  Bus Selector4/1 -> Derivative8/1  "<x>"
  Bus Selector4/2 -> Derivative9/1  "<y>"
  Derivative8/1 -> MATLAB Function6/1(vx)  "vx"
  Derivative9/1 -> MATLAB Function6/2(vy)  "vy"
  Derivative6/1 -> MATLAB Function5/1(vx)  "vx"
  Gazebo Read3/2 -> Bus Selector1/1
  Bus Selector1/1 -> Derivative6/1  "<x>"
  Bus Selector1/2 -> Derivative7/1  "<y>"
  Gazebo Read4/2 -> Bus Selector4/1
  Derivative7/1 -> MATLAB Function5/2(vy)  "vy"
  MATLAB Function5/1(v) -> Sum/1, Gain/1  "v_L"
  Gain/1 -> w_L/1  "w_L"
  MATLAB Function6/1(v) -> Sum/2, Gain1/1  "v_R"
  Gain1/1 -> w_R/1  "w_R"
  Sum/1 -> Gain2/1
  Gain2/1 -> v_car/1

== system full_system/Torque control/Apply left wheel torque ==
  torque : Inport  SampleTime=0.001
  Bus Assignment : BusAssignment  AssignedSignals=model_name,joint_name,index,effort,duration.nano_seconds
  Constant : Constant  Value=0  OutDataTypeStr=uint32  SampleTime=0.001
  Constant1 : Constant  Value=1e7  SampleTime=0.001
  Gazebo Apply Command : robotgazebolib/Gazebo Apply Command  cmdType=ApplyJointTorque  sampleTime=0.001
  Gazebo Blank Message : robotgazebolib/Gazebo Blank Message  msgType=ApplyJointTorque  sampleTime=0.001  busName='Gazebo_SL_Bus_gazebo_msgs_ApplyJointTorque'
  Gazebo Select Entity : robotgazebolib/Gazebo Select Entity  modelElemName=pioneer2dx/left_wheel_hinge  outputArraySize=128  OutputLabel=Joint  SelectType=Joint
  wires:
  Gazebo Select Entity/1 -> Bus Assignment/2
  Bus Assignment/1 -> Gazebo Apply Command/1
  Gazebo Blank Message/1 -> Bus Assignment/1
  Constant/1 -> Bus Assignment/4
  Gazebo Select Entity/2 -> Bus Assignment/3
  Constant1/1 -> Bus Assignment/6
  torque/1 -> Bus Assignment/5

== system full_system/Torque control/Apply right wheel torque ==
  torque : Inport  SampleTime=0.001
  Bus Assignment : BusAssignment  AssignedSignals=model_name,joint_name,index,effort,duration.nano_seconds
  Constant : Constant  Value=0  OutDataTypeStr=uint32  SampleTime=0.001
  Constant1 : Constant  Value=1e7  SampleTime=0.001
  Gazebo Apply Command : robotgazebolib/Gazebo Apply Command  cmdType=ApplyJointTorque  sampleTime=0.001
  Gazebo Blank Message : robotgazebolib/Gazebo Blank Message  msgType=ApplyJointTorque  sampleTime=0.001  busName='Gazebo_SL_Bus_gazebo_msgs_ApplyJointTorque'
  Gazebo Select Entity : robotgazebolib/Gazebo Select Entity  modelElemName=pioneer2dx/right_wheel_hinge  outputArraySize=128  OutputLabel=Joint  SelectType=Joint
  wires:
  Gazebo Select Entity/1 -> Bus Assignment/2
  Bus Assignment/1 -> Gazebo Apply Command/1
  Gazebo Blank Message/1 -> Bus Assignment/1
  Constant/1 -> Bus Assignment/4
  Gazebo Select Entity/2 -> Bus Assignment/3
  Constant1/1 -> Bus Assignment/6
  torque/1 -> Bus Assignment/5

== matlab function full_system/get actual wheel speeds2/MATLAB Function5 ==
  settings: updateMethod=DISCRETE
  data: vx input; v output; vy input
function v = detSpeed(vx, vy)
persistent prev_x
persistent prev_y

if isempty(prev_x)
    prev_x = 0;
end

if isempty(prev_y)
    prev_y = 0;
end

if abs(prev_x - vx)>1
    vx = prev_x;
else
    prev_x = vx;
end

if abs(prev_y - vy)>1
    vy = prev_y;
else 
    prev_y = vy;
end

v = sqrt(vx^2 + vy^2);

== matlab function full_system/get actual wheel speeds2/MATLAB Function6 ==
  settings: updateMethod=DISCRETE
  data: vx input; v output; vy input
function v = detSpeed(vx, vy)
persistent prev_x
persistent prev_y

if isempty(prev_x)
    prev_x = 0;
end

if isempty(prev_y)
    prev_y = 0;
end

if abs(prev_x - vx)>1
    vx = prev_x;
else
    prev_x = vx;
end

if abs(prev_y - vy)>1
    vy = prev_y;
else 
    prev_y = vy;
end

v = sqrt(vx^2 + vy^2);

== matlab function full_system/Measure wheel speeds/MATLAB Function6 ==
  settings: updateMethod=DISCRETE
  data: vx input; v output; vy input
function v = detSpeed(vx, vy)
persistent prev_x
persistent prev_y

if isempty(prev_x)
    prev_x = 0;
end

if isempty(prev_y)
    prev_y = 0;
end

if abs(prev_x - vx)>1
    vx = prev_x;
else
    prev_x = vx;
end

if abs(prev_y - vy)>1
    vy = prev_y;
else 
    prev_y = vy;
end

v = sqrt(vx^2 + vy^2);

== matlab function full_system/get actual wheel speeds3/MATLAB Function5 ==
  settings: updateMethod=DISCRETE
  data: vx input; v output; vy input
function v = detSpeed(vx, vy)
persistent prev_x
persistent prev_y

if isempty(prev_x)
    prev_x = 0;
end

if isempty(prev_y)
    prev_y = 0;
end

if abs(prev_x - vx)>1
    vx = prev_x;
else
    prev_x = vx;
end

if abs(prev_y - vy)>1
    vy = prev_y;
else 
    prev_y = vy;
end

v = sqrt(vx^2 + vy^2);

== matlab function full_system/get actual wheel speeds3/MATLAB Function6 ==
  settings: updateMethod=DISCRETE
  data: vx input; v output; vy input
function v = detSpeed(vx, vy)
persistent prev_x
persistent prev_y

if isempty(prev_x)
    prev_x = 0;
end

if isempty(prev_y)
    prev_y = 0;
end

if abs(prev_x - vx)>1
    vx = prev_x;
else
    prev_x = vx;
end

if abs(prev_y - vy)>1
    vy = prev_y;
else 
    prev_y = vy;
end

v = sqrt(vx^2 + vy^2);

== matlab function full_system/calc torques1/MATLAB Function ==
  data: in_L input; out_L output; in_R input; out_R output
function [out_L, out_R] = checkMinDiff(in_L, in_R)
min_diff = 0.005;

if abs(in_L)>=min_diff
    out_L = in_L;
else
    out_L = 0;
end

if abs(in_R)>=min_diff
    out_R = in_R;
else
    out_R = 0;
end

== matlab function full_system/Torque control/MATLAB Function ==
  data: in_L input; out_L output; in_R input; out_R output
function [out_L, out_R] = checkMinDiff(in_L, in_R)
min_diff = 0.005;

if abs(in_L)>=min_diff
    out_L = in_L;
else
    out_L = 0;
end

if abs(in_R)>=min_diff
    out_R = in_R;
else
    out_R = 0;
end

== matlab function full_system/MATLAB Function2 ==
  data: angle output; s_node input; t_node input; x input; y input; base_speed input; speed output; targetReached output; dist_to_next output; seg output
function [angle, speed, targetReached, dist_to_next, seg] = getRoute(s_node, t_node, x, y, base_speed)
persistent routePlanner
persistent segment_num
persistent reached_target
coder.extrinsic("route_planner")
coder.extrinsic("get_ref_array")

brake_point = 0.5; %distance from t_node where braking should start
node_radius = 0.1; 

if isempty(reached_target)
    reached_target = 0;
end

xt = 0;
yt = 0;
len = 0;
angle = 0;
speed = 0;

%speed = base_speed;

%

if isempty(routePlanner)
    routePlanner = route_planner();
end

if isempty(segment_num)
    segment_num = 1;
end

ref_signal = get_ref_array(routePlanner, s_node, t_node);
len = size(ref_signal,2);

xt = ref_signal(3, segment_num);
yt = ref_signal(4, segment_num);

if reached_target==0
    speed = base_speed;
    angle = atan((yt-y)/(xt-x));
end

dist_to_next = sqrt((yt-y)^2 + (xt-x)^2);

if (segment_num==len)&&(dist_to_next<=brake_point)&&(reached_target==0)
    speed = base_speed*dist_to_next/brake_point;
end

seg = segment_num;

if dist_to_next < node_radius
    if (segment_num==len)
        %segment_num = 1;
        reached_target = 1;
    else
        segment_num = segment_num+1;
    end
end

targetReached = reached_target;

== matlab function full_system/Measure car pose/MATLAB Function ==
  data: in input; out output
function out = correctAngle(in)
% out = wrapTo2Pi(in);
persistent prev_angle

if isempty(prev_angle)
    prev_angle = 0;
end
% % 
% % temp = unwrap([0, in]);
% % out = temp(2);
% % prev_angle = out;
% % if in<0
% %     in = in+2*pi;
% % end
% % 
% % if in>2*pi
% %     out = in-2*pi;
% % else
% %     out=in;
% % end

temp = unwrap([prev_angle, in]);
out = temp(2);
out = wrapTo2Pi(out);
prev_angle = out;
% temp = unwrap([0, in], (2*pi));
% in = temp(2);
% prev_angle = in;
% out = in;

== matlab function full_system/Camera stuff/find markers ==
  data: frame input; id output; loc output; pose output; gotMarker output; x output; y output
function [id, loc, pose, gotMarker, x, y] = findMarkers(frame) % [status, id, loc, pose, gotMarker] = findMarkers(frame, params)
% persistent intrinsics
% coder.extrinsic('readAprilTag')
% 
% status = 0;     % 0 : params empty | 1 : params not empty
% tag_family = "tag36h11";
% tag_size = 0.1; %10cm
% 
% id = 0;
% loc = 0;
% pose = 0;
% gotMarker = 0;
% 
% disp(size(frame))
% 
% if isempty(intrinsics)&&(~isempty(params))
% 
%     focal_length = params(1:2);
%     principal_point = params(3:4);
%     image_size = [2464, 3280]; %params(5:6);
%     radial_distortion = params(7:8);
% 
%     intrinsics = cameraIntrinsics(focal_length, ...
%         principal_point, image_size, 'RadialDistortion', ...
%         radial_distortion);
% 
% end
% 
% if ~isempty(intrinsics)
%     frame = undistortImage(frame, intrinsics, OutputView='same');
%     [id, loc, pose] = readAprilTag(frame, tag_family, intrinsics, tag_size);
% 
%     if isempty(loc)
%         gotMarker = 0;
%     else
%         gotMarker = 1;
%     end
% end
% 
% if ~isempty(params)
%     status = 1;
% end


persistent cam_helper
coder.extrinsic("camHelper")
coder.extrinsic("getMarkers")

max_markers = 1;
id = 404; % zeros(max_markers, 1, 1);
loc = zeros(4, 2, 1);
pose = zeros(4, 4, 1);
%pose = rigidtform3d(A);
x = 0;
y = 0;

gotMarker = 0;

if isempty(cam_helper)
    cam_helper = camHelper;
end

[id, loc, pose, gotMarker, x, y] = getMarkers(cam_helper, frame);

== matlab function full_system/Camera stuff/MATLAB Function ==
  data: data input; processed_data output
function processed_data=processVideo(data)
% the camera sends a 1200*600*3 data signal. Simulink receives it as a 1-D
% array

width = 3280;
height = 2464;
z = 3;

processed_data = zeros(height, width, z, 'uint8');

if ~isempty(data) && ~isscalar(data)

    indexBase = (1:z:width*height*z)';
    index = zeros(numel(indexBase), z);

    for i=1:z
        index(:, i) = indexBase + i - 1;
    end

    temp = reshape(data(index), width, height, z);
    processed_data = permute(temp, [2 1 3]);

end

== matlab function full_system/MATLAB Function1 ==
  data: targetReached output; angle output; s_node input; t_node input; x input; y input; base_speed input; speed output
function [targetReached, angle, speed] = getRoute(s_node, t_node, x, y, base_speed)
persistent routePlanner
persistent segment_num
persistent reached_target
coder.extrinsic("route_planner")
coder.extrinsic("get_ref_array")

brake_point = 0.5; %distance from t_node where braking should start
node_radius = 0.1; 

if isempty(reached_target)
    reached_target = 0;
end


xt = 0;
yt = 0;
len = 0;
angle = 0;
speed = 0;

if isempty(routePlanner)
    routePlanner = route_planner();
end

if isempty(segment_num)
    segment_num = 1;
end

ref_signal = get_ref_array(routePlanner, s_node, t_node);
len = size(ref_signal,2);

xt = ref_signal(3, segment_num);
yt = ref_signal(4, segment_num);


speed = base_speed;
angle = atan((yt-y)/(xt-x));

% if xt<x
%     angle = pi+angle;
% end
% 
% error_angle = angle-meas_angle;
% 
% if error_angle>pi
%     error_angle = -error_angle;
% end

dist_to_next = sqrt((yt-y)^2 + (xt-x)^2);

if (segment_num==len)&&(dist_to_next<=brake_point)&&(reached_target==0)
    speed = base_speed*dist_to_next/brake_point;
end

if dist_to_next < node_radius
    if (segment_num==len)
        %segment_num = 1;
        reached_target = 1;
    else
        segment_num = segment_num+1;
    end
end

targetReached = reached_target;

== matlab function full_system/Measure wheel speeds/MATLAB Function5 ==
  settings: updateMethod=DISCRETE
  data: vx input; v output; vy input
function v = detSpeed(vx, vy)
persistent prev_x
persistent prev_y

if isempty(prev_x)
    prev_x = 0;
end

if isempty(prev_y)
    prev_y = 0;
end

if abs(prev_x - vx)>1
    vx = prev_x;
else
    prev_x = vx;
end

if abs(prev_y - vy)>1
    vy = prev_y;
else 
    prev_y = vy;
end

v = sqrt(vx^2 + vy^2);

== matlab function full_system/get actual wheel speeds/MATLAB Function5 ==
  settings: updateMethod=DISCRETE
  data: vx input; v output; vy input
function v = detSpeed(vx, vy)
persistent prev_x
persistent prev_y

if isempty(prev_x)
    prev_x = 0;
end

if isempty(prev_y)
    prev_y = 0;
end

if abs(prev_x - vx)>1
    vx = prev_x;
else
    prev_x = vx;
end

if abs(prev_y - vy)>1
    vy = prev_y;
else 
    prev_y = vy;
end

v = sqrt(vx^2 + vy^2);

== matlab function full_system/get actual wheel speeds/MATLAB Function6 ==
  settings: updateMethod=DISCRETE
  data: vx input; v output; vy input
function v = detSpeed(vx, vy)
persistent prev_x
persistent prev_y

if isempty(prev_x)
    prev_x = 0;
end

if isempty(prev_y)
    prev_y = 0;
end

if abs(prev_x - vx)>1
    vx = prev_x;
else
    prev_x = vx;
end

if abs(prev_y - vy)>1
    vy = prev_y;
else 
    prev_y = vy;
end

v = sqrt(vx^2 + vy^2);

== matlab function full_system/get actual wheel speeds1/MATLAB Function5 ==
  settings: updateMethod=DISCRETE
  data: vx input; v output; vy input
function v = detSpeed(vx, vy)
persistent prev_x
persistent prev_y

if isempty(prev_x)
    prev_x = 0;
end

if isempty(prev_y)
    prev_y = 0;
end

if abs(prev_x - vx)>1
    vx = prev_x;
else
    prev_x = vx;
end

if abs(prev_y - vy)>1
    vy = prev_y;
else 
    prev_y = vy;
end

v = sqrt(vx^2 + vy^2);

== matlab function full_system/get actual wheel speeds1/MATLAB Function6 ==
  settings: updateMethod=DISCRETE
  data: vx input; v output; vy input
function v = detSpeed(vx, vy)
persistent prev_x
persistent prev_y

if isempty(prev_x)
    prev_x = 0;
end

if isempty(prev_y)
    prev_y = 0;
end

if abs(prev_x - vx)>1
    vx = prev_x;
else
    prev_x = vx;
end

if abs(prev_y - vy)>1
    vy = prev_y;
else 
    prev_y = vy;
end

v = sqrt(vx^2 + vy^2);
